simulink model "bamboo_lam"  (R2022b)
settings: Solver=VariableStepAuto  StartTime=0.0  StopTime=1800  RelTol=1e-3
libraries: VACLib x7
settings Model: Creator=KarlO  LastModifiedBy=KOQVIST1

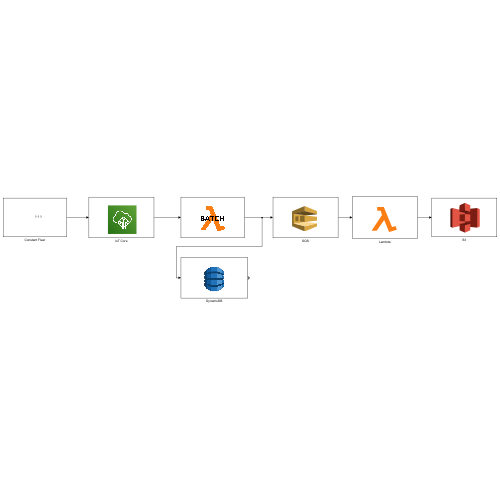
[thumbnail: Simulink's stored preview of the top-level diagram]
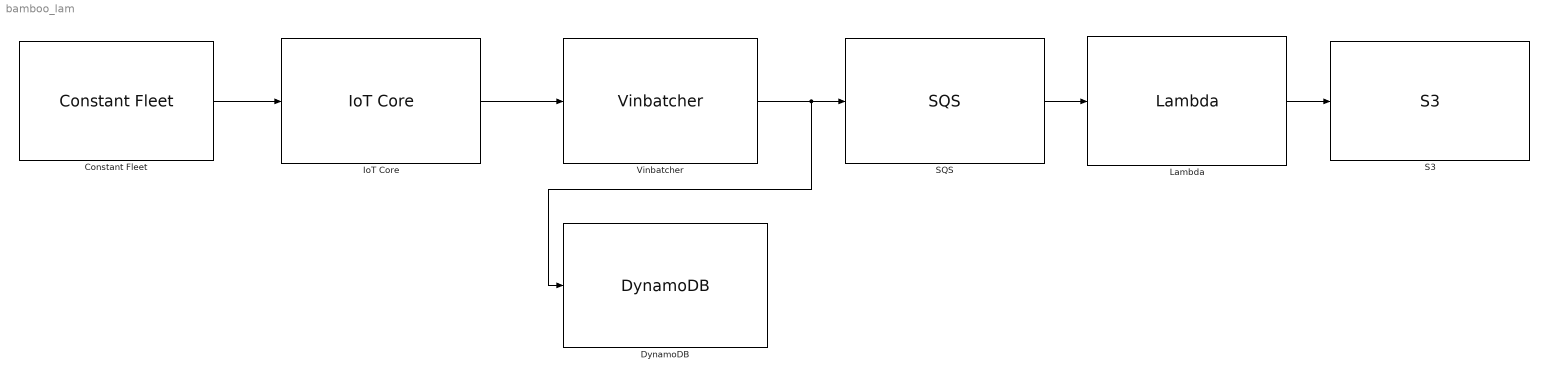
== system bamboo_lam ==
  Constant Fleet : VACLib/Vehicle Components/Constant Fleet  SystemSampleTime=-1  VariantActivationTime=update diagram  Latency=0  AutoFrameSizeCalculation=off
      settings: SourceProductName=Volvo Architechture Components
  DynamoDB : VACLib/AWS Components/DynamoDB  SystemSampleTime=-1  VariantActivationTime=update diagram  Latency=0  AutoFrameSizeCalculation=off
      settings: SourceProductName=Volvo Architechture Components
  IoT Core : VACLib/AWS Components/IoT Core  SystemSampleTime=-1  VariantActivationTime=update diagram  Latency=0  AutoFrameSizeCalculation=off
      settings: SourceProductName=Volvo Architechture Components
  Lambda : VACLib/AWS Components/Lambda  SystemSampleTime=-1  VariantActivationTime=update diagram  Latency=0  AutoFrameSizeCalculation=off
      settings: SourceProductName=Volvo Architechture Components
  S3 : VACLib/AWS Components/S3  SystemSampleTime=-1  VariantActivationTime=update diagram  Latency=0  AutoFrameSizeCalculation=off
      settings: SourceProductName=Volvo Architechture Components
  SQS : VACLib/AWS Components/SQS  SystemSampleTime=-1  VariantActivationTime=update diagram  Latency=0  AutoFrameSizeCalculation=off
      settings: SourceProductName=Volvo Architechture Components
  Vinbatcher : VACLib/AWS Components/Vinbatcher  SystemSampleTime=-1  VariantActivationTime=update diagram  Latency=0  AutoFrameSizeCalculation=off
      settings: SourceProductName=Volvo Architechture Components
  wires:
  IoT Core/1 -> Vinbatcher/1
  Vinbatcher/1 -> SQS/1, DynamoDB/1
  SQS/1 -> Lambda/1
  Lambda/1 -> S3/1
  Constant Fleet/1 -> IoT Core/1
